simulink model "aaa1"  (R2021b)
settings: Solver=VariableStepAuto  StartTime=0.0  StopTime=3  RelTol=1e-3
libraries: simulink x2
settings Model: Creator=郭义月  LastModifiedBy=郭义月

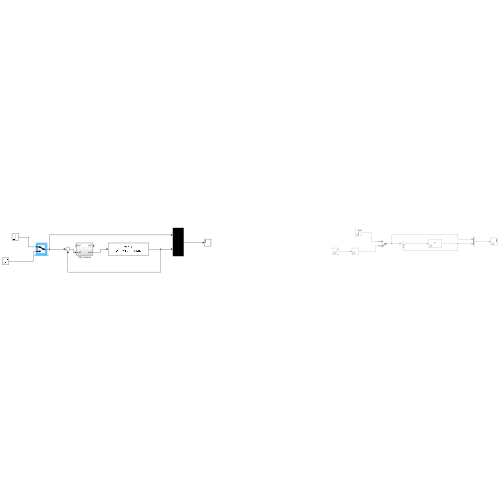
[thumbnail: Simulink's stored preview of the top-level diagram]
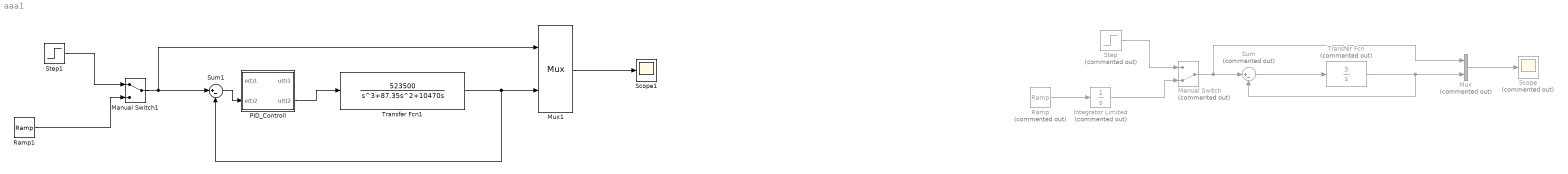
== system aaa1 ==
  Integrator Limited : Integrator  Commented=on  LimitOutput=on  UpperSaturationLimit=1000  LowerSaturationLimit=0
  Manual Switch : ManualSwitch  Commented=on  CurrentSetting=0
  Manual Switch1 : ManualSwitch
  Mux : Mux  Commented=on  Inputs=2
  Mux1 : Mux  Inputs=2
  PID_Controll : Subsystem
  Ramp : simulink/Sources/Ramp  Commented=on  slope=1  start=0  InitialOutput=0
  Ramp1 : simulink/Sources/Ramp  slope=1  start=0  InitialOutput=0
  Scope : Scope  Commented=on
  Scope1 : Scope
  Step : Step  Commented=on  SampleTime=0
  Step1 : Step  SampleTime=0
  Sum : Sum  Commented=on  Inputs=|+-
  Sum1 : Sum  Inputs=|+-
  Transfer Fcn : TransferFcn  Commented=on  Numerator=[3]  Denominator=[1 0]
  Transfer Fcn1 : TransferFcn  Numerator=[523500]  Denominator=[1 87.35 10470 0]
  wires:
  Step/1 -> Manual Switch/1
  Ramp/1 -> Integrator Limited/1
  Sum/1 -> Transfer Fcn/1
  Transfer Fcn/1 -> Mux/2, Sum/2
  Mux/1 -> Scope/1
  Manual Switch/1 -> Mux/1, Sum/1
  Step1/1 -> Manual Switch1/1
  Manual Switch1/1 -> Sum1/1, Mux1/1
  Transfer Fcn1/1 -> Mux1/2, Sum1/2
  Mux1/1 -> Scope1/1
  Integrator Limited/1 -> Manual Switch/2
  Ramp1/1 -> Manual Switch1/2
  Sum1/1 -> PID_Controll/2(e(t)2)
  PID_Controll/2(u(t)2) -> Transfer Fcn1/1

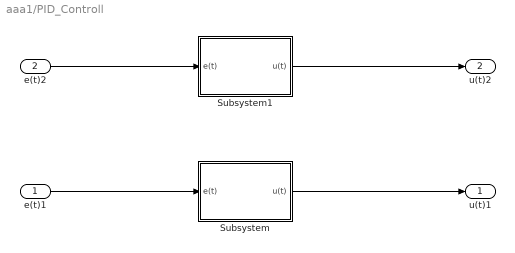
== system aaa1/PID_Controll ==
  e(t)1 : Inport
  e(t)2 : Inport  Port=2
  Subsystem : Subsystem
  Subsystem1 : Subsystem
  u(t)1 : Outport
  u(t)2 : Outport  Port=2
  wires:
  e(t)1/1 -> Subsystem/1(e(t))
  Subsystem/1(u(t)) -> u(t)1/1
  Subsystem1/1(u(t)) -> u(t)2/1
  e(t)2/1 -> Subsystem1/1(e(t))

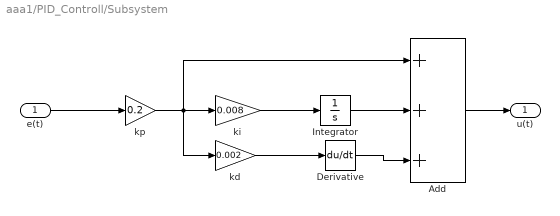
== system aaa1/PID_Controll/Subsystem ==
  e(t) : Inport
  Add : Sum  Inputs=+++
  Derivative : Derivative
  Integrator : Integrator
  kd : Gain  Gain=0.002
  ki : Gain  Gain=0.008
  kp : Gain  Gain=0.2
  u(t) : Outport
  wires:
  Integrator/1 -> Add/2
  Add/1 -> u(t)/1
  kd/1 -> Derivative/1
  e(t)/1 -> kp/1
  kp/1 -> Add/1, kd/1, ki/1
  ki/1 -> Integrator/1
  Derivative/1 -> Add/3

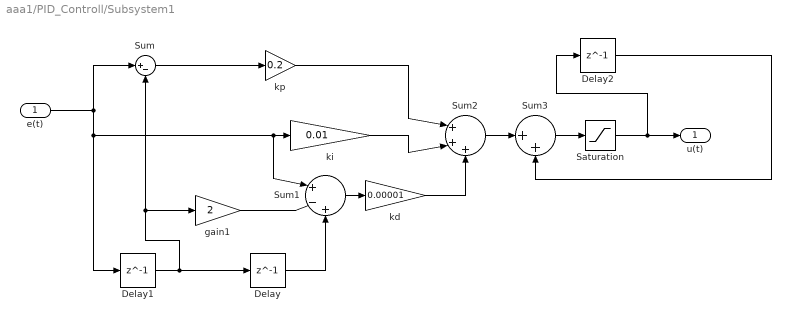
== system aaa1/PID_Controll/Subsystem1 ==
  e(t) : Inport
  Delay : Delay  DelayLength=1  InitialCondition=0
  Delay1 : Delay  DelayLength=1  InitialCondition=0
  Delay2 : Delay  DelayLength=1  InitialCondition=0
  Saturation : Saturate
  Sum : Sum  Inputs=|+-
  Sum1 : Sum  Inputs=|+-+
  Sum2 : Sum  Inputs=|+++
  Sum3 : Sum  Inputs=|++
  gain1 : Gain  Gain=2
  kd : Gain  Gain=0.00001
  ki : Gain  Gain=0.01
  kp : Gain  Gain=0.2
  u(t) : Outport
  wires:
  Sum2/1 -> Sum3/1
  e(t)/1 -> Sum/1, Delay1/1, Sum1/1, ki/1
  Sum/1 -> kp/1
  kp/1 -> Sum2/1
  Sum3/1 -> Saturation/1
  Saturation/1 -> Delay2/1, u(t)/1
  Delay2/1 -> Sum3/2
  ki/1 -> Sum2/2
  Delay1/1 -> Delay/1, Sum/2, gain1/1
  Delay/1 -> Sum1/3
  Sum1/1 -> kd/1
  kd/1 -> Sum2/3
  gain1/1 -> Sum1/2
